simulink model "lab0_2"  (R2021a)
settings: Solver=VariableStepAuto  StartTime=0.0  StopTime=10.0  RelTol=1e-3
settings Model: Creator=Giancarlo  LastModifiedBy=Giancarlo

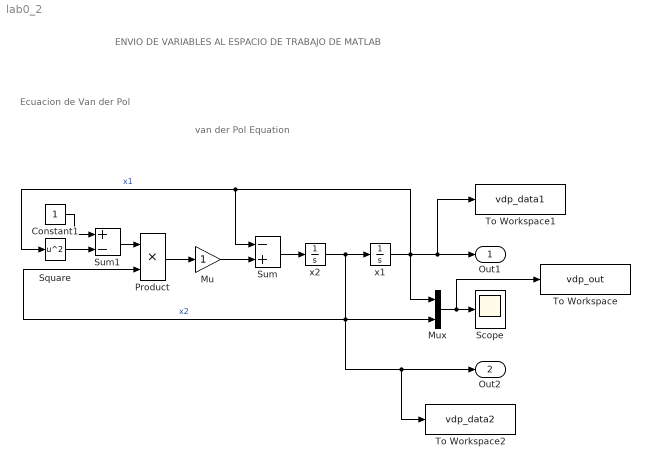
== system lab0_2 ==
  note: Ecuacion de Van der Pol
  note: ENVIO DE VARIABLES AL ESPACIO DE TRABAJO DE MATLAB
  note: van der Pol Equation
  Constant1 : Constant
  Mu : Gain  SaturateOnIntegerOverflow=on  OutDataTypeStr=Inherit: Same as input  ParamDataTypeStr=Inherit: Same as input
  Mux : Mux  Inputs=2
  Product : Product  InputSameDT=on  RndMeth=Zero  SaturateOnIntegerOverflow=on  OutDataTypeStr=Inherit: Same as first input
  Scope : Scope
  Square : Math  Operator=square  SaturateOnIntegerOverflow=on
  Sum : Sum  Inputs=-+  InputSameDT=on  SaturateOnIntegerOverflow=on  OutDataTypeStr=Inherit: Same as first input
  Sum1 : Sum  Inputs=+-  InputSameDT=on  SaturateOnIntegerOverflow=on  OutDataTypeStr=Inherit: Same as first input
  To Workspace : ToWorkspace  VariableName=vdp_out  SampleTime=-1
  To Workspace1 : ToWorkspace  VariableName=vdp_data1  SampleTime=-1
  To Workspace2 : ToWorkspace  VariableName=vdp_data2  SampleTime=-1
  x1 : Integrator  InitialCondition=1
  x2 : Integrator  InitialCondition=1
  Out1 : Outport  InitialOutput=0  VectorParamsAs1DForOutWhenUnconnected=off
  Out2 : Outport  Port=2  InitialOutput=0  VectorParamsAs1DForOutWhenUnconnected=off
  wires:
  x2/1 -> To Workspace2/1, Out2/1, Mux/2, Product/2, x1/1  "x2"
  Mu/1 -> Sum/2
  Sum/1 -> x2/1
  Sum1/1 -> Product/1
  Constant1/1 -> Sum1/1
  Product/1 -> Mu/1
  Mux/1 -> To Workspace/1, Scope/1
  x1/1 -> To Workspace1/1, Out1/1, Mux/1, Square/1, Sum/1  "x1"
  Square/1 -> Sum1/2
